simulink model "Clutchless_P2_Parallel_ETE"  (R2017b)
settings: Solver=FixedStepAuto  StartTime=0.0  StopTime=length(Speed)  FixedStep=0.01  MaxStep=0.01  RelTol=1e-3  EnableMultiTasking=on
PostLoadFcn:
  | , if any(exist('dsrtsu_mdlpostloadfcn', 'file') == [2, 3, 6]), try dsrtsu_mdlpostloadfcn('Execute', bdroot); catch fprintf('Error in PostLoadFcn (dsrtsu_mdlpostloadfcn) for model "%s":\n %s\n', bdroot, lasterr); end, end,
undefined symbols (not defined in the file): ABSEnable, Actuators, air, APP1_OOR, APP2_OOR, APP_Mismatch, Brk_Flt, cal, ClutchEngag, Clutchless_HSC_ETE, CS_On_Control, Driver, eng, Engine, EngOverTemp, ENGTRQ_MSMCH_Degraded_CP, ENGTRQ_MSMCH_ErrCritical_CP, ENGTRQ_MSMCH_LimpHome_CP, EngTrqMismatch, env, ess, ESSOverTemp, gb, KeyPos_Flt, KeyPosition, lib_Actuators, lib_Clutchless_HSC_ETE, lib_Driver, lib_EMachine_2017a, lib_Sensors_2017a, LossCAN, Machine, max_vehicle_rad_air_flow, MCUOverTemp, mot, MotDirMismatch, MotOverTemp, MotTrqMismatch, mph2ms, PRNDL_Flt, RegenBrkDisable, RegenFault, Sensors, ShiftLeverPosition, Speed, SW_CS_ON, SW_Engine_ON, t_amb, time, tloop
libraries: simulink x97, Pneumatic_lib x11, nesl_utility x9, EC2_libraries x7, powerlib_meascontrol x2, CalculationGallon x1, lib_Chassis x1, lib_DCDC x1, lib_Differential x1, lib_HVESS x1, fl_lib x1, lib_OBC x1
(part 1 of 9)
settings Model: DSRTSU_INTERNAL_RTI_VER=480  DSRTSU_INTERNAL_RTI_TYPE=rti1006  RTICANMMDATA=struct('GeneralSetupData',struct('modelroot','D:\EcoCAR3\Controls\HIL\Y3\P2_Parallel_MIL_Model','generalsettings',struct('filesettings',struct('destfolder',struct('Name','RTICANMM_FILES','Check',1),'buildfolder',struct('Name','.','Check',1),'AbsDestfolder',struct('Name','D:\EcoCAR3\Controls\HIL\Y3\P2_Parallel_MIL_Model\RTICANMM_FILES'),'AbsBuildfolder',struct('Name','D:\EcoCAR3\Controls\HIL\Y3\P2_Parallel_MIL_Model'))),'options',struct('addpaths',1,'rmpaths',1,'addtrcexclusion',logical(1),'cannavigator',struct('checkmonitoring',0),'show_usrtrc',0,'use_usrtrc',0),'advanced',struct('options',[1 1 1 1 1 1 1 1 1 1 1 1 1 1 1 1 1 1 1 1 1 1 1 1 1 1 1 1 1 1 1 1 1 1 1 1 1 1 1 1 1 1 1 1 1 1 1 1 1 1 1 1 1 1 1 1 1 1 1 1 1 1 1 1 1 1 1 1 1 1 1 1 1 1 1 1 1 1 1 1 1 1 1 1 1 1 1 1 1 1 1 1 1 1 1 1 1 1 1 1]),'MPSetup',{{}},'modelname','P2_Parallel_MIL_02_16_2017','block','P2_Parallel_MIL_02_16_2017'))  DSRTSU_INTERNAL_RTIFPGA=70  SimulationMode=accelerator  Creator=EcoCar  LastModifiedBy=Lyu19
settings SolverCC: ExtrapolationOrder=1  NumberNewtonIterations=4
settings OptimizationCC: BlockReduction=off  OptimizeBlockIOStorage=off  BufferReuse=off  GlobalBufferReuse=off  ExpressionFolding=off  LocalBlockOutputs=off  EfficientMapNaN2IntZero=off
settings DebuggingCC: AllowSymbolicDim=off  NonBusSignalsTreatedAsBus=warning  SFUnexpectedBacktrackingDiag=warning  SFNoUnconditionalDefaultTransitionDiag=warning  SFExecutionAtInitializationDiag=none
settings HardwareCC: ProdBitPerPointer=32  ProdBitPerSizeT=32  ProdBitPerPtrDiffT=32  ProdLargestAtomicInteger=Integer  ProdWordSize=32  ProdHWDeviceType=Custom Processor->Custom  TargetBitPerPointer=64  TargetBitPerSizeT=64  TargetBitPerPtrDiffT=64  TargetLongLongMode=on  TargetIntDivRoundTo=Zero  TargetEndianess=LittleEndian  TargetWordSize=64  TargetHWDeviceType=MATLAB Host  ProdEqTarget=off
settings ModelReferenceCC: PropagateSignalLabelsOutOfModel=off
settings CodeAppCC: MaxIdLength=128  StateflowObjectComments=on
settings GRTTargetCC: TargetLangStandard=C89/C90 (ANSI)  CombineOutputUpdateFcns=off  GRTInterface=on
settings ConfigComp: CovMetricSettings=dw  CovHtmlReporting=on  CovSaveCumulativeToWorkspaceVar=on  CovSaveSingleToWorkspaceVar=on  CovExternalEMLEnable=off
settings SimscapeCC: SimscapeNormalizeSystem=off

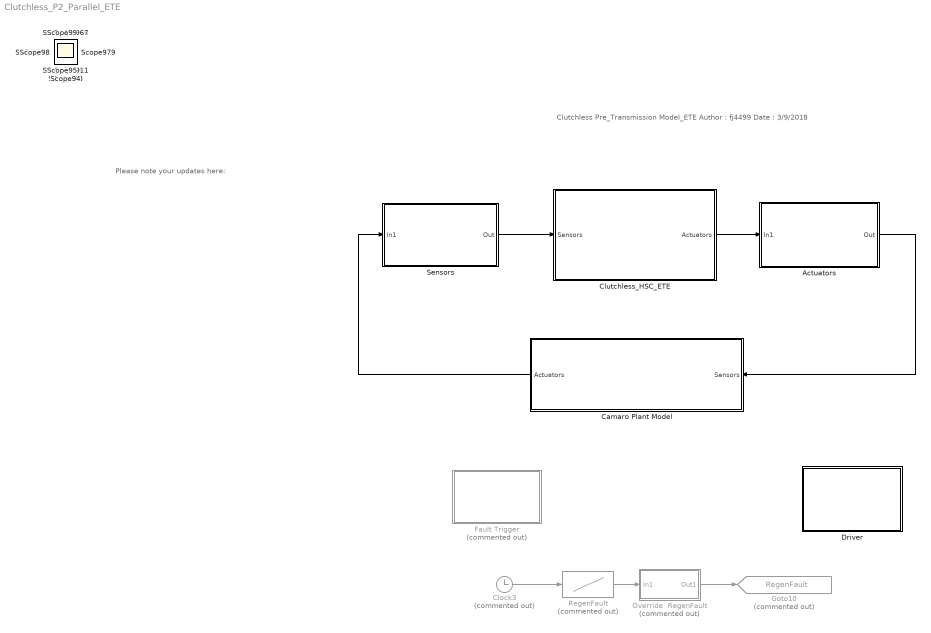
== system Clutchless_P2_Parallel_ETE ==
  note: Please note your updates here:
  note: Clutchless Pre_Transmission Model_ETE
      |
      | Author : fj4499
      | Date : 3/9/2018
  Actuators : Subsystem  AncestorBlock=lib_Actuators/Actuators
  Camaro Plant Model : Subsystem
      mask Display: image('Images/Vehicle.jpg')
  Clock3 : Clock  Commented=on
  Clutchless_HSC_ETE : Subsystem  AncestorBlock=lib_Clutchless_HSC_ETE/Clutchless_HSC_ETE
      mask Display: image('Images/HCU.jpg')
  Driver : Subsystem  AncestorBlock=lib_Driver/Driver
      mask Display: image('Images/Driver.jpg')
  "Fault Trigger " : Subsystem  Commented=on  mask(Fault Trigger){Mismatch_APP_ON=on, APP1_OOR_ON=on, APP2_OOR_ON=on, Brk_Flt_ON=on, KeyPos_Flt_ON=on, PRNDL_Flt_ON=on, LossCAN_ON=on, MotTrqMismatch_ON=on, MotDirMismatch_ON=on, EngTrqMismatch_ON=on, MotOverTemp_ON=on, MCUOverTemp_ON=on, EngOverTemp_ON=on, ESSOverTemp_ON=on, ClutchEngagFlt=on}
      mask help:
      | Check the box: override the fault (Control Port value=1;)
      | Uncheck the box: Implement the fault (Control Port value=0;)
      mask DialogControl DriverInterfaceFault Prompt: Driver Interface Fault
      mask DialogControl Container3 Prompt: Component Fault
      mask Display:
      | plot([1 2 2.01 3 4], [0 0 1 1 1]);
      | disp('           Fault Trigger')
  Goto10 : Goto  Commented=on  GotoTag=RegenFault  TagVisibility=global
  Override  RegenFault : Subsystem  Commented=on
  RegenFault : Lookup  Commented=on  InputValues=time  Table=RegenFault  LookUpMeth=Interpolation-Use End Values  OutDataTypeStr=int8
  Sensors : Subsystem  AncestorBlock=lib_Sensors_2017a/Sensors
  Scope{,1..141} (142 alike) : Scope
  wires:
  Clock3/1 -> RegenFault/1
  RegenFault/1 -> Override  RegenFault/1(In1)
  Override  RegenFault/1(Out1) -> Goto10/1
  Clutchless_HSC_ETE/1(Actuators) -> Actuators/1(In1)
  Actuators/1(Out) -> Camaro Plant Model/1(Sensors)
  Camaro Plant Model/1(Actuators) -> Sensors/1(In1)
  Sensors/1(Out) -> Clutchless_HSC_ETE/1(Sensors)

== system Clutchless_P2_Parallel_ETE/Actuators ==
  In1 : Inport
  Analog : Subsystem
  Bus Creator : BusCreator  Inputs=3
  CAN : Subsystem
  Digital : Subsystem
  Memory : Memory  InheritSampleTime=on
  Out : Outport
  wires:
  In1/1 -> CAN/1(In1), Analog/1(In1), Digital/1(In1)
  Bus Creator/1 -> Memory/1
  Digital/1(Out1) -> Bus Creator/3  "Digital"
  CAN/1(Out1) -> Bus Creator/1  "CAN"
  Analog/1(Out1) -> Bus Creator/2  "Analog"
  Memory/1 -> Out/1

== system Clutchless_P2_Parallel_ETE/Camaro Plant Model ==
  Sensors : Inport
  Add : Sum  Inputs=+++
      mask Display:
      | port_label('input',1,'+');
      | port_label('input',2,'+');
      | port_label('input',3,'+');
  Bus Creator : BusCreator  Inputs=3
  Bus Creator1 : BusCreator  Inputs=7
  Bus Creator2 : BusCreator  Inputs=1
  Bus Selector : BusSelector  OutputSignals=Analog,CAN.to VEH_CAN,CAN.to EBCAN,CAN.to HV_CAN,Digital
  Calculate MPGe : CalculationGallon/Calculate MPGe
  Chassis : lib_Chassis/Chassis  SystemSampleTime=-1
      link override Grade: InputValues=time
  DC-DC Converter : lib_DCDC/DC-DC Converter  SystemSampleTime=-1
  Differential : lib_Differential/Differential  SystemSampleTime=-1
      settings: SourceProductName=The database C:\Users\vrajm\AppData\Roaming\MathWorks\MATLAB\R2017b\slblocks_master.db is locked, or a table in the database is locked. (database is locked)
  E-Machine : Subsystem  AncestorBlock=lib_EMachine_2017a/E-Machine
      mask Display:
      | image('Images/motor.png')
      | color('red');
      | port_label('Input',1,'Volt');
      | port_label('Input',2,'ShaftIn');
      | port_label('Input',3,'SpdOut');
      | port_label('Output',1,'Crr');
      | port_label('Output',2,'ShaftOut');
      | port_label('Output',3,'SpdIn');
  ESS : lib_HVESS/ESS  SystemSampleTime=-1
  Ground : Ground
  ICE Simple1 : Subsystem  AncestorBlock=lib_Engine/ICE Simple1
      mask Display:
      | image(imread('EngineTopLevel.jpg'),'center')
      | color('red');
      | port_label('input',1,'SpdOut')
      | port_label('output',1,'ShaftOut')
  On-Board Charger : lib_OBC/On-Board Charger  SystemSampleTime=-1
      settings: SourceProductName=The database C:\Users\vrajm\AppData\Roaming\MathWorks\MATLAB\R2017b\slblocks_master.db is locked, or a table in the database is locked. (database is locked)
  Scopes : Subsystem  Commented=on
      mask Display: image('Images/Scope.jpg')
  Scopes1 : Scope_new/Scopes1  SystemSampleTime=-1
  Transmission : lib_Transmission/Transmission  SystemSampleTime=-1
  Transmission Validation Results : Transmission_Validation/Transmission Validation Results  Commented=on  SystemSampleTime=-1
  Wheels : lib_Wheels/Wheels  SystemSampleTime=-1
      link override Grade: InputValues=time
      settings: SourceProductName=The database C:\Users\vrajm\AppData\Roaming\MathWorks\MATLAB\R2017b\slblocks_master.db is locked, or a table in the database is locked. (database is locked)
  Actuators : Outport
  tag scope: Analog=global, Digital=global, HCU_to_EBCAN=global, HCU_to_HV_CAN=global, HCU_to_VEH_CAN=global
  wires:
  Differential/1 -> Wheels/1
  Wheels/1 -> Chassis/1
  Chassis/1 -> Wheels/2
  Differential/2 -> Transmission/2
  Transmission/1 -> Differential/1
  ESS/1 -> DC-DC Converter/1, E-Machine/1(voltage), On-Board Charger/1
  DC-DC Converter/1 -> Add/3
  On-Board Charger/1 -> Add/2
  Add/1 -> ESS/1
  Transmission/2 -> E-Machine/3(Mot_SpdOut)
  E-Machine/2(Motor_ShaftOut) -> Transmission/1
  E-Machine/1(current) -> Add/1
  Bus Creator/1 -> Actuators/1
  Sensors/1 -> Bus Selector/1
  Bus Selector/1 -> [Analog]  "<Analog>"
  Bus Selector/2 -> [HCU_to_VEH_CAN]  "<to VEH_CAN>"
  Bus Selector/3 -> [HCU_to_EBCAN]  "<to EBCAN>"
  Bus Selector/4 -> [HCU_to_HV_CAN]  "<to HV_CAN>"
  Bus Selector/5 -> [Digital]  "<Digital>"
  Wheels/2 -> Differential/2
  E-Machine/3(Motor_SpdIn) -> ICE Simple1/1(eng_spd_out)
  [ECM_to_HCU] -> Bus Creator1/1
  [TCM_to_HCU] -> Bus Creator1/2
  [BCM_to_HCU] -> Bus Creator1/3
  [BMS_to_HCU] -> Bus Creator1/4
  [MCU_to_HCU] -> Bus Creator1/5
  Bus Creator2/1 -> Bus Creator1/6  "APM_to_HCU"
  [OBC_to_HCU] -> Bus Creator1/7
  Bus Creator1/1 -> Bus Creator/1  "CAN"
  [Driver_Request] -> Bus Creator/2  "Driver_Signals"
  [DCDC_to_HCU] -> Bus Creator/3
  Ground/1 -> Bus Creator2/1  "APM_CAN"
  ICE Simple1/1(eng_shaft_out) -> E-Machine/2(Mot_ShaftIn)

== system Clutchless_P2_Parallel_ETE/Clutchless_HSC_ETE ==
  Sensors : Inport
  HSC : Subsystem
  Actuators : Outport
  wires:
  Sensors/1 -> HSC/1(Sensors)
  HSC/1(Actuators) -> Actuators/1

== system Clutchless_P2_Parallel_ETE/Driver ==
  Bus Creator : BusCreator  Inputs=12
  Bus Selector : BusSelector  OutputSignals=GFD_Light,HV_Chg_Light,Veh_Ready_Light
  Constant : Constant  Commented=on  Value=0
  Display : Display
  Display1 : Display
  Display2 : Display
  Driver Control : Subsystem
  Manual Control : Subsystem  Commented=on
  Multiport Switch1 : MultiPortSwitch  Commented=on  DataPortOrder=Zero-based contiguous  Inputs=2
  Subsystem : Subsystem
  tag scope: Driver_Request=global
  wires:
  Driver Control/11(Sport_Mode_SW) -> Bus Creator/12  "Sport_Mode_SW"
  Driver Control/10(ABS_Active) -> Bus Creator/11  "ABSAtv"
  Subsystem/2(APP2) -> Bus Creator/3
  Subsystem/1(APP1) -> Bus Creator/2
  Bus Selector/3 -> Display2/1  "<Veh_Ready_Light>"
  Bus Selector/2 -> Display1/1  "<HV_Chg_Light>"
  Bus Selector/1 -> Display/1  "<GFD_Light>"
  [Digital] -> Bus Selector/1
  Driver Control/9(CS_On) -> Bus Creator/10  "SW_CS_ON"
  Driver Control/8(Engine_On) -> Bus Creator/9  "SW_Engine_ON"
  Driver Control/7(Regen_Disable) -> Bus Creator/8  "SW_Regen_Disable"
  Driver Control/6(Veh_Spd) -> Bus Creator/7  "Veh_Spd"
  Bus Creator/1 -> [Driver_Request]
  Manual Control/1(Out1) -> Multiport Switch1/3
  Constant/1 -> Multiport Switch1/1
  Driver Control/5(EVSE_Pluggin) -> Bus Creator/6  "EVSE_Plugged"
  Driver Control/4(Shift Lever Position) -> Bus Creator/5  "ShiftLvrPos"
  Driver Control/3(BPP[%]) -> Bus Creator/4  "drv_BPP_req_[%]"
  Driver Control/2(APP[%]) -> Subsystem/1(In1)  "drv_APP_req_[%]"
  Driver Control/1(Key Position) -> Bus Creator/1  "KeyPos"

== system Clutchless_P2_Parallel_ETE/Fault Trigger  ==
  Clock3 : Clock
  Component Diagnostics setting : Subsystem
  Driver Interface Diagnostics setting : Subsystem
  wires:
  Clock3/1 -> Component Diagnostics setting/1(time), Driver Interface Diagnostics setting/1(time)

== system Clutchless_P2_Parallel_ETE/Override  RegenFault ==
  note: This subsystem is used to override the model value of a signal to a constant value
  note: Override Switch Subsystem
  In1 : Inport
  Constant : Constant  Value=0
  Multiport Switch : MultiPortSwitch  DataPortOrder=Zero-based contiguous  Inputs=2
  Signal Override Switch 0 = Use Model 1 = Use Constant : Constant  Value=0
  Out1 : Outport
  wires:
  Signal Override Switch 0 = Use Model 1 = Use Constant/1 -> Multiport Switch/1
  In1/1 -> Multiport Switch/2
  Multiport Switch/1 -> Out1/1
  Constant/1 -> Multiport Switch/3

== system Clutchless_P2_Parallel_ETE/Sensors ==
  In1 : Inport
  Analog : Subsystem
  Bus Creator : BusCreator  Inputs=3
  Bus Selector : BusSelector  OutputSignals=CAN
  CAN : Subsystem
  Digital : Subsystem
  Out : Outport
  wires:
  Bus Creator/1 -> Out/1
  In1/1 -> Digital/1(In1), Analog/1(In1), Bus Selector/1
  Bus Selector/1 -> CAN/1(In1)  "<CAN>"
  CAN/1(Out1) -> Bus Creator/1  "from_CAN"
  Analog/1(Out1) -> Bus Creator/2  "from_Analog"
  Digital/1(Out1) -> Bus Creator/3  "from_Digital"

== system Clutchless_P2_Parallel_ETE/Actuators/Analog ==
  In1 : Inport
  Bus Creator : BusCreator  Inputs=1
  Bus Selector : BusSelector  OutputSignals=Controls.EngAppReq
  Data Type Conversion : DataTypeConversion
  Out1 : Outport
  wires:
  In1/1 -> Bus Selector/1
  Bus Creator/1 -> Out1/1
  Bus Selector/1 -> Data Type Conversion/1  "<EngAppReq>"
  Data Type Conversion/1 -> Bus Creator/1  "EngAppReq"

== system Clutchless_P2_Parallel_ETE/Actuators/CAN ==
  In1 : Inport
  Bus Creator : BusCreator  Inputs=3
  EBCAN : Subsystem
  HV_CAN : Subsystem
  VEH_CAN : Subsystem
  Out1 : Outport
  wires:
  VEH_CAN/1(Out1) -> Bus Creator/1  "to VEH_CAN"
  EBCAN/1(Out1) -> Bus Creator/2  "to EBCAN"
  HV_CAN/1(Out1) -> Bus Creator/3  "to HV_CAN"
  Bus Creator/1 -> Out1/1
  In1/1 -> HV_CAN/1(In1), EBCAN/1(In1), VEH_CAN/1(In1)

== system Clutchless_P2_Parallel_ETE/Actuators/Digital ==
  In1 : Inport
  Bus Creator : BusCreator  Inputs=8
  Bus Selector : BusSelector  OutputSignals=BMS_Digital.T_15,BMS_Digital.T_30,BMS_Digital.T_30C,Fuel_Pump_Control.Pump_Commands.FuelPump_Disable,OBC_Digital.Brusa_Enable,Axiomatic_CAN.GFD_Light,Axiomatic_CAN.HV_Chg_Light,Axiomatic_CAN.Veh_Ready_Light
  Data Type Conversion : DataTypeConversion
  Data Type Conversion1 : DataTypeConversion
  Out1 : Outport
  wires:
  In1/1 -> Bus Selector/1
  Bus Creator/1 -> Out1/1  "Digital"
  Bus Selector/4 -> Bus Creator/4  "<FuelPump_Disable>"
  Bus Selector/3 -> Bus Creator/3  "<T_30C>"
  Bus Selector/2 -> Data Type Conversion1/1  "<T_30>"
  Bus Selector/1 -> Data Type Conversion/1  "<T_15>"
  Bus Selector/5 -> Bus Creator/5  "<Brusa_Enable>"
  Bus Selector/6 -> Bus Creator/6  "<GFD_Light>"
  Bus Selector/7 -> Bus Creator/7  "<HV_Chg_Light>"
  Bus Selector/8 -> Bus Creator/8  "<Veh_Ready_Light>"
  Data Type Conversion/1 -> Bus Creator/1  "T_15"
  Data Type Conversion1/1 -> Bus Creator/2  "T_30"

== system Clutchless_P2_Parallel_ETE/Camaro Plant Model/E-Machine ==
  voltage : Inport
  Mot_ShaftIn : Inport  Port=2
  Mot_SpdOut : Inport  Port=3
  Clutch Temporary 1 : Subsystem  Commented=on
  IMG Plant : Subsystem
      mask Display:
      | image('Images\Motor.png')
      | color('red');
      | port_label('Input',2,'Volt');
      | port_label('Input',3,'ShaftIn');
      | port_label('Input',4,'SpdOut');
      | port_label('Output',2,'Crr');
      | port_label('Output',3,'ShaftOut');
      | port_label('Output',4,'SpdIn');
  IMG Plant2 : Subsystem  Commented=on
      mask Display:
      | image('Images/motor.png')
      | color('red');
      | port_label('Input',2,'Volt');
      | port_label('Input',3,'SpdOut');
      | port_label('Input',1,'MCU_cmd');
      | port_label('Input',4,'ShaftIn');
      | port_label('Output',1,'Sensor_Out');
      | port_label('Output',2,'Crr');
      | port_label('Output',3,'MotTrqOut');
      | port_label('Output',4,'MotSpdIn');
  Soft MCU : Subsystem
      mask Display: image('SoftECU.jpg')
  current : Outport
  Motor_ShaftOut : Outport  Port=2
  Motor_SpdIn : Outport  Port=3
  tag scope: MCU_to_HCU=global
  wires:
  IMG Plant/2(current) -> current/1
  voltage/1 -> IMG Plant/2(voltage)
  IMG Plant/3(MotShaftOut) -> Motor_ShaftOut/1
  Mot_ShaftIn/1 -> IMG Plant/3(MotShaftIn)
  IMG Plant/1(Out1) -> Soft MCU/2(In1)  "Sensors_to_MCU"
  [HCU_to_HV_CAN] -> Soft MCU/1(In)
  Soft MCU/2(Out1) -> IMG Plant/1("In1 ")  "MCU_to_Actuators"
  Soft MCU/1(Out) -> [MCU_to_HCU]
  Mot_SpdOut/1 -> IMG Plant/4(SpdOut)
  IMG Plant/4(SpdIn) -> Motor_SpdIn/1

== system Clutchless_P2_Parallel_ETE/Camaro Plant Model/ICE Simple1 ==
  eng_spd_out : Inport
  Engine Plant Modified : Subsystem
      mask Display:
      | image(imread('EngineTopLevel.jpg'),'center')
      | color('red');
      | port_label('input',2,'SpdOut')
      | port_label('output',2,'ShaftOut')
  Inputs : Subsystem
  Soft ECM : Subsystem
      mask Display: image('SoftECU.jpg')
  eng_shaft_out : Outport
  tag scope: ECM_to_HCU=global
  wires:
  Engine Plant Modified/2(Out) -> Soft ECM/2(In1)
  eng_spd_out/1 -> Engine Plant Modified/2(eng_spd_out)
  Soft ECM/2(Out1) -> Engine Plant Modified/1("In ")  "ECM_to_Actuators"
  Inputs/1(Inputs) -> Soft ECM/1(In)
  Soft ECM/1(Out) -> [ECM_to_HCU]
  Engine Plant Modified/1(eng_shaft_out) -> eng_shaft_out/1

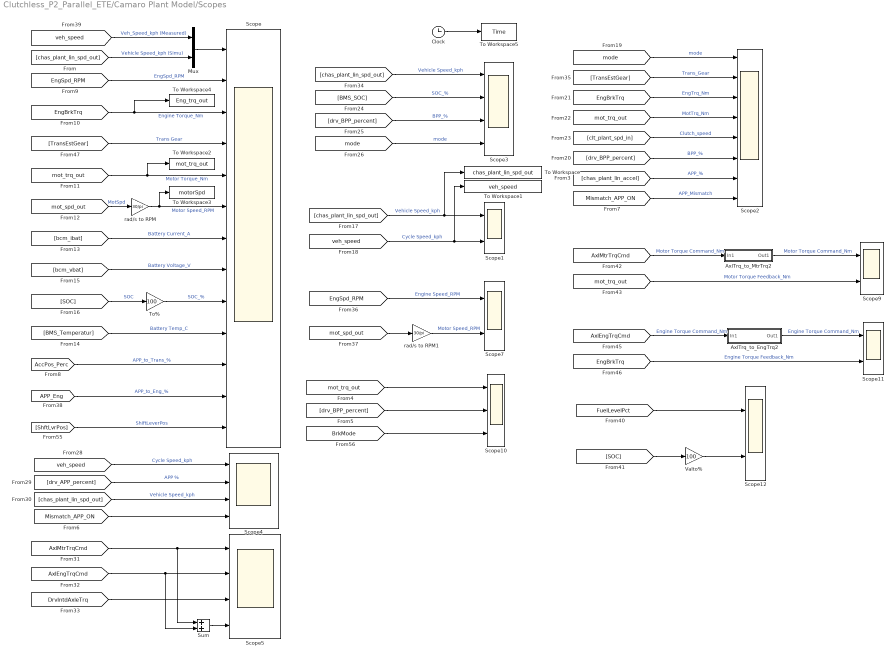
== system Clutchless_P2_Parallel_ETE/Camaro Plant Model/Scopes ==
  AxlTrq_to_EngTrq2 : Subsystem
  AxlTrq_to_MtrTrq2 : Subsystem
  Clock : Clock
      settings: Decimation=WORKSPACE_DECIMATION
  Mux : Mux  Inputs=2
  Scope : Scope  NumInputPorts=13
  Scope{1,7,9,11..12} (5 alike) : Scope  NumInputPorts=2
  Scope10 : Scope  NumInputPorts=3
  Scope2 : Scope  NumInputPorts=8
  Scope3 : Scope  NumInputPorts=4
  Scope4 : Scope  NumInputPorts=4
  Scope5 : Scope  NumInputPorts=4
  Sum : Sum
  To Workspace : ToWorkspace  VariableName=chas_plant_lin_spd_out  SampleTime=-1
  To Workspace1 : ToWorkspace  VariableName=veh_speed  SampleTime=-1
  To Workspace2 : ToWorkspace  VariableName=mot_trq_out  SampleTime=-1
  To Workspace3 : ToWorkspace  VariableName=motorSpd  SampleTime=-1
  To Workspace4 : ToWorkspace  VariableName=Eng_trq_out  SampleTime=-1
  To Workspace5 : ToWorkspace  VariableName=Time  SampleTime=-1
      settings: Decimation=WORKSPACE_DECIMATION
  To% : Gain  Gain=100
  Valto% : Gain  Gain=100
  rad/s to RPM : Gain  Gain=30/pi
  rad/s to RPM1 : Gain  Gain=30/pi
  wires:
  [chas_plant_lin_spd_out] -> Mux/2  "Vehicle Speed_kph (Simu)"
  [EngSpd_RPM] -> Scope/2  "EngSpd_RPM"
  [EngBrkTrq] -> To Workspace4/1, Scope/3  "Engine Torque_Nm"
  [mot_spd_out] -> rad/s to RPM/1  "MotSpd"
  [BMS_Temperatur] -> Scope/10  "Battery Temp_C"
  rad/s to RPM/1 -> To Workspace3/1, Scope/6  "Motor Speed_RPM"
  [mot_trq_out] -> To Workspace2/1, Scope/5  "Motor Torque_Nm"
  To%/1 -> Scope/9  "SOC_%"
  [TransEstGear] -> Scope/4  "Trans Gear"
  [bcm_ibat] -> Scope/7  "Battery Current_A"
  [chas_plant_lin_spd_out] -> Scope3/1  "Vehicle Speed_kph"
  [BMS_SOC] -> Scope3/2  "SOC_%"
  [drv_BPP_percent] -> Scope3/3  "BPP_%"
  [mode] -> Scope3/4  "mode"
  [chas_plant_lin_spd_out] -> To Workspace/1, Scope1/1  "Vehicle Speed_kph"
  [veh_speed] -> To Workspace1/1, Scope1/2  "Cycle Speed_kph"
  [mode] -> Scope2/1  "mode"
  [EngBrkTrq] -> Scope2/3  "EngTrq_Nm"
  [mot_trq_out] -> Scope2/4  "MotTrq_Nm"
  [clt_plant_spd_in] -> Scope2/5  "Clutch_speed"
  [EngSpd_RPM] -> Scope7/1  "Engine Speed_RPM"
  [mot_spd_out] -> rad/s to RPM1/1
  rad/s to RPM1/1 -> Scope7/2  "Motor Speed_RPM"
  [veh_speed] -> Scope4/1  "Cycle Speed_kph"
  [drv_APP_percent] -> Scope4/2  "APP %"
  [chas_plant_lin_spd_out] -> Scope4/3  "Vehicle Speed_kph"
  [AxlMtrTrqCmd] -> Sum/1, Scope5/1
  [AxlEngTrqCmd] -> Sum/2, Scope5/2
  [DrvIntdAxleTrq] -> Scope5/3
  Sum/1 -> Scope5/4
  [AxlMtrTrqCmd] -> AxlTrq_to_MtrTrq2/1(In1)  "Motor Torque Command_Nm"
  [mot_trq_out] -> Scope9/2  "Motor Torque Feedback_Nm"
  [AxlEngTrqCmd] -> AxlTrq_to_EngTrq2/1(In1)  "Engine Torque Command_Nm"
  [EngBrkTrq] -> Scope11/2  "Engine Torque Feedback_Nm"
  [TransEstGear] -> Scope2/2  "Trans_Gear"
  [drv_BPP_percent] -> Scope2/6  "BPP_%"
  [chas_plant_lin_accel] -> Scope2/7  "APP_%"
  AxlTrq_to_MtrTrq2/1(Out1) -> Scope9/1  "Motor Torque Command_Nm"
  AxlTrq_to_EngTrq2/1(Out1) -> Scope11/1  "Engine Torque Command_Nm"
  [bcm_vbat] -> Scope/8  "Battery Voltage_V"
  [Mismatch_APP_ON] -> Scope4/4
  [Mismatch_APP_ON] -> Scope2/8  "APP_Mismatch"
  [SOC] -> To%/1  "SOC"
  [AccPos_Perc] -> Scope/11  "APP_to_Trans_%"
  [APP_Eng] -> Scope/12  "APP_to_Eng_%"
  Mux/1 -> Scope/1
  [veh_speed] -> Mux/1  "Veh_Speed_kph (Measured)"
  Clock/1 -> To Workspace5/1
  [FuelLevelPct] -> Scope12/1
  [SOC] -> Valto%/1
  Valto%/1 -> Scope12/2
  [ShftLvrPos] -> Scope/13  "ShiftLeverPos"
  [mot_trq_out] -> Scope10/1
  [drv_BPP_percent] -> Scope10/2
  [BrkMode] -> Scope10/3

== system Clutchless_P2_Parallel_ETE/Clutchless_HSC_ETE/HSC ==
  Sensors : Inport
  Camaro Fault Detection : Subsystem
  Driver_Requests : Subsystem  RequirementInfo={} %GIDa_ee5d0f02_0a71_4952_8ea3_2a40744828e3
  Powertrain Manager : Subsystem
  Actuators : Outport
  wires:
  Powertrain Manager/2(Controls) -> Driver_Requests/3("Controls ")
  Sensors/1 -> Camaro Fault Detection/1(Sensors), Powertrain Manager/1(Sensors), Driver_Requests/1(Sensors)
  Powertrain Manager/1(Out1) -> Actuators/1
  Camaro Fault Detection/1(Diagnostic) -> Powertrain Manager/3(Fault Detection), Driver_Requests/2("Diagnostic ")
  Driver_Requests/1(DriverRequests) -> Powertrain Manager/2(Driver Request)

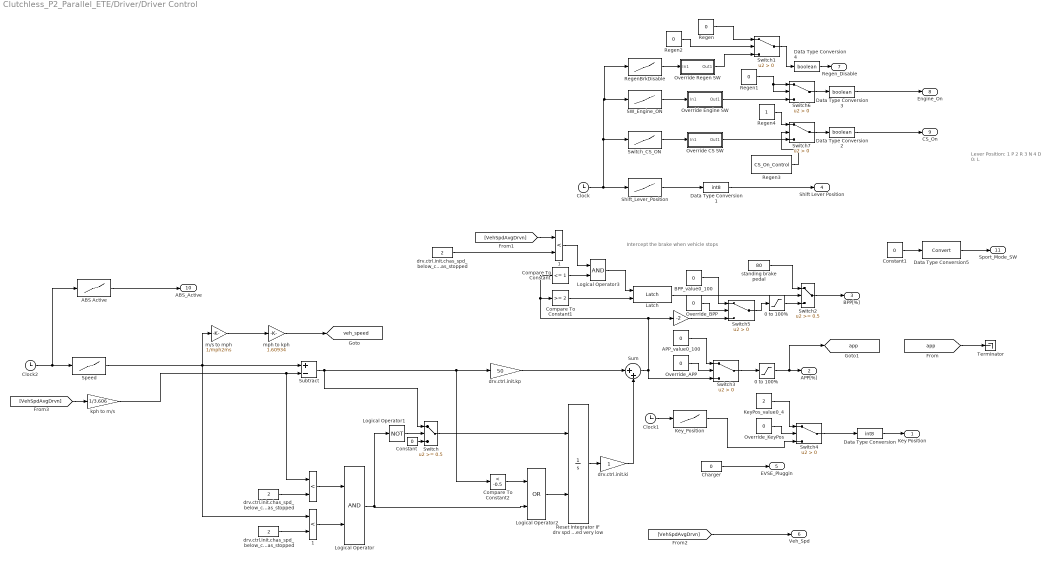
== system Clutchless_P2_Parallel_ETE/Driver/Driver Control ==
  note: Intercept the brake when vehicle stops
  note: Lever Position:
      | 1 P
      | 2 R
      | 3 N
      | 4 D
      | 0: L
  " " : Gain  Gain=-2
  "    " : RelationalOperator  Operator=<  RndMeth=Nearest  InputSameDT=on
  "    1" : RelationalOperator  Operator=<  RndMeth=Nearest  InputSameDT=on
  "  1" : RelationalOperator  Operator=<  RndMeth=Nearest  InputSameDT=on
  0 to 100% : Saturate  UpperLimit=100  LowerLimit=0
  "0 to 100% " : Saturate  UpperLimit=100  LowerLimit=0
  ABS Active : Lookup  InputValues=time  Table=ABSEnable
  APP_value0_100 : Constant  Value=0
  BPP_value0_100 : Constant  Value=0
  Charger : Constant  Value=0
  Clock : Clock
  Clock1 : Clock
  Clock2 : Clock
  Compare To Constant : simulink/Logic and Bit Operations/Compare To Constant  relop=<=  const=1  OutDataTypeStr=boolean
  Compare To Constant1 : simulink/Logic and Bit Operations/Compare To Constant  relop=>=  const=2  OutDataTypeStr=boolean
  Compare To Constant2 : simulink/Logic and Bit Operations/Compare To Constant  relop=<  const=-0.5  OutDataTypeStr=boolean
  Constant : Constant  Value=0
  Constant1 : Constant  Value=0
  Data Type Conversion : DataTypeConversion  OutDataTypeStr=int8
  Data Type Conversion1 : DataTypeConversion  OutDataTypeStr=int8
  Data Type Conversion2 : DataTypeConversion  OutDataTypeStr=boolean
  Data Type Conversion3 : DataTypeConversion  OutDataTypeStr=boolean
  Data Type Conversion4 : DataTypeConversion  OutDataTypeStr=boolean
  Data Type Conversion5 : DataTypeConversion
  KeyPos_value0_4 : Constant  Value=2
  Key_Position : Lookup  InputValues=time  Table=KeyPosition
  Latch : Utility/Latch
  Logical Operator : Logic  AllPortsSameDT=off  OutDataTypeStr=boolean
  Logical Operator1 : Logic  Operator=NOT  AllPortsSameDT=off  OutDataTypeStr=boolean
  Logical Operator2 : Logic  Operator=OR  AllPortsSameDT=off  OutDataTypeStr=boolean
  Logical Operator3 : Logic  AllPortsSameDT=off  OutDataTypeStr=boolean
  Override CS SW : Subsystem
  Override Engine SW : Subsystem
  Override Regen SW : Subsystem
  Override_APP : Constant  Value=0
  Override_BPP : Constant  Value=0
  Override_KeyPos : Constant  Value=0
  Regen : Constant  Value=0
  Regen1 : Constant  Value=0
  Regen2 : Constant  Value=0
  Regen3 : Constant  Value=CS_On_Control
  Regen4 : Constant
  RegenBrkDisable : Lookup  InputValues=time  Table=RegenBrkDisable
  Reset Integrator IF drv spd dmd very low AND AND current vehicle speed very low : Integrator  ExternalReset=either
  SW_Engine_ON : Lookup  InputValues=time  Table=SW_Engine_ON
  Shift_Lever_Position : Lookup  InputValues=time  Table=ShiftLeverPosition
  Speed : Lookup  InputValues=time  Table=Speed
  Subtract : Sum  Inputs=+-
  Sum : Sum  Inputs=|++  SaturateOnIntegerOverflow=on  InputSameDT=on  OutDataTypeStr=Inherit: Same as first input
  Switch : Switch  Threshold=0.5
  Switch{1,3..7} (6 alike) : Switch  Criteria=u2 > Threshold
  Switch2 : Switch  Threshold=0.5
  Switch_CS_ON : Lookup  InputValues=time  Table=SW_CS_ON
  Terminator : Terminator
  "drv.ctrl.init.chas_spd_below_chas_stopped " : Constant  Value=2
  "drv.ctrl.init.chas_spd_below_chas_stopped " : Constant  Value=2
  "drv.ctrl.init.chas_spd_below_chas_stopped " : Constant  Value=2
  drv.ctrl.init.ki : Gain  SaturateOnIntegerOverflow=on  OutDataTypeStr=Inherit: Same as input  ParamDataTypeStr=Inherit: Same as input
  drv.ctrl.init.kp : Gain  Gain=50  SaturateOnIntegerOverflow=on  OutDataTypeStr=Inherit: Same as input  ParamDataTypeStr=Inherit: Same as input
  kph to m/s : Gain  Gain=1/3.606  SaturateOnIntegerOverflow=on  OutDataTypeStr=Inherit: Same as input  ParamDataTypeStr=Inherit: Same as input
  m/s to mph : Gain  Gain=1/mph2ms
  mph to kph : Gain  Gain=1.60934
  standing brake pedal : Constant  Value=80
  Key Position : Outport
  APP[%] : Outport  Port=2
  BPP[%] : Outport  Port=3
  Shift Lever Position : Outport  Port=4
  EVSE_Pluggin : Outport  Port=5
  Veh_Spd : Outport  Port=6
  Regen_Disable : Outport  Port=7
  Engine_On : Outport  Port=8
  CS_On : Outport  Port=9
  ABS_Active : Outport  Port=10
  Sport_Mode_SW : Outport  Port=11
  tag scope: app=global, veh_speed=global
  wires:
  Speed/1 -> "  1"/1, m/s to mph/1, Subtract/1
  [app] -> Terminator/1
  Regen4/1 -> Switch7/1
  Regen3/1 -> Switch7/2
  Override CS SW/1(Out1) -> Switch7/3
  Switch7/1 -> Data Type Conversion2/1
  Regen2/1 -> Switch1/2
  Constant1/1 -> Data Type Conversion5/1
  Data Type Conversion5/1 -> Sport_Mode_SW/1
  ABS Active/1 -> ABS_Active/1
  kph to m/s/1 -> "    "/1, Subtract/2
  Switch6/1 -> Data Type Conversion3/1
  Override Engine SW/1(Out1) -> Switch6/3
  Data Type Conversion3/1 -> Engine_On/1
  Regen1/1 -> Switch6/1, Switch6/2
  Switch1/1 -> Data Type Conversion4/1
  Regen/1 -> Switch1/1
  Shift_Lever_Position/1 -> Data Type Conversion1/1
  Switch5/1 -> "0 to 100% "/1
  BPP_value0_100/1 -> Switch5/1
  Override_BPP/1 -> Switch5/2
  Latch/1 -> Switch2/2
  Switch4/1 -> Data Type Conversion/1
  KeyPos_value0_4/1 -> Switch4/1
  Override_KeyPos/1 -> Switch4/2
  Key_Position/1 -> Switch4/3
  APP_value0_100/1 -> Switch3/1
  Override_APP/1 -> Switch3/2
  Switch3/1 -> 0 to 100%/1
  [VehSpdAvgDrvn] -> Veh_Spd/1
  Data Type Conversion4/1 -> Regen_Disable/1
  Data Type Conversion2/1 -> CS_On/1
  Override Regen SW/1(Out1) -> Switch1/3
  RegenBrkDisable/1 -> Override Regen SW/1(In1)
  SW_Engine_ON/1 -> Override Engine SW/1(In1)
  Switch_CS_ON/1 -> Override CS SW/1(In1)
  0 to 100%/1 -> APP[%]/1, [app]
  mph to kph/1 -> [veh_speed]
  m/s to mph/1 -> mph to kph/1
  Clock2/1 -> Speed/1, ABS Active/1
  Clock1/1 -> Key_Position/1
  Clock/1 -> Shift_Lever_Position/1, Switch_CS_ON/1, SW_Engine_ON/1, RegenBrkDisable/1
  Compare To Constant2/1 -> Logical Operator2/1
  Subtract/1 -> Switch/1, drv.ctrl.init.kp/1, Compare To Constant2/1
  Charger/1 -> EVSE_Pluggin/1
  Data Type Conversion1/1 -> Shift Lever Position/1
  Data Type Conversion/1 -> Key Position/1
  Compare To Constant1/1 -> Latch/2
  Compare To Constant/1 -> Logical Operator3/2
  Logical Operator3/1 -> Latch/1
  Sum/1 -> Switch3/3, " "/1, Compare To Constant/1, Compare To Constant1/1
  "    1"/1 -> Logical Operator3/1
  "drv.ctrl.init.chas_spd_below_chas_stopped "/1 -> "    1"/2
  [VehSpdAvgDrvn] -> "    1"/1
  Switch2/1 -> BPP[%]/1
  standing brake pedal/1 -> Switch2/1
  [VehSpdAvgDrvn] -> kph to m/s/1
  " "/1 -> Switch5/3
  "0 to 100% "/1 -> Switch2/3
  Logical Operator/1 -> Logical Operator1/1, Logical Operator2/2
  "  1"/1 -> Logical Operator/2
  drv.ctrl.init.ki/1 -> Sum/2
  "drv.ctrl.init.chas_spd_below_chas_stopped "/1 -> "  1"/2
  Logical Operator2/1 -> Reset Integrator IF drv spd dmd very low AND AND current vehicle speed very low/2
  Switch/1 -> Reset Integrator IF drv spd dmd very low AND AND current vehicle speed very low/1
  "drv.ctrl.init.chas_spd_below_chas_stopped "/1 -> "    "/2
  Logical Operator1/1 -> Switch/2
  Reset Integrator IF drv spd dmd very low AND AND current vehicle speed very low/1 -> drv.ctrl.init.ki/1
  Constant/1 -> Switch/3
  "    "/1 -> Logical Operator/1
  drv.ctrl.init.kp/1 -> Sum/1

== system Clutchless_P2_Parallel_ETE/Driver/Manual Control ==
  note: Manipulate these values
      | to drive vehicle
  APP[%] : Constant
  BPP[%] : Constant  Value=-1
  Bus Creator1 : BusCreator  Inputs=5
  KeyPosition : Constant  Value=3
  PRNDL : Constant  Value=4
  ReferenceVel1 : Constant  Value=0
  Saturation : Saturate  UpperLimit=100  LowerLimit=0
  Saturation1 : Saturate  UpperLimit=0  LowerLimit=-100
  Saturation2 : Saturate  UpperLimit=3  LowerLimit=0
  Saturation3 : Saturate  UpperLimit=4  LowerLimit=0
  Slider Gain : simulink/Math Operations/Slider Gain  gain=0  low=0  high=100
  Slider Gain1 : simulink/Math Operations/Slider Gain  gain=0  low=0  high=100
  Out1 : Outport
  wires:
  Slider Gain1/1 -> Saturation1/1
  Slider Gain/1 -> Saturation/1
  Saturation3/1 -> Bus Creator1/4  "PRNDL"
  PRNDL/1 -> Saturation3/1
  ReferenceVel1/1 -> Bus Creator1/5  "refVel [m/s]"
  APP[%]/1 -> Slider Gain/1
  BPP[%]/1 -> Slider Gain1/1
  Bus Creator1/1 -> Out1/1  "DriverOut"
  KeyPosition/1 -> Saturation2/1
  Saturation/1 -> Bus Creator1/1  "APP (%)"
  Saturation1/1 -> Bus Creator1/2  "BPP(%)"
  Saturation2/1 -> Bus Creator1/3  "Key_Pos_[0_3]"

== system Clutchless_P2_Parallel_ETE/Driver/Subsystem ==
  In1 : Inport
  Add1 : Sum  Inputs=+++
  Add2 : Sum
  Constant1 : Constant  Value=0
  Constant2 : Constant  Value=cal.APP.Mismatch_Value+0.1
  Constant3 : Constant  Value=0
  Constant4 : Constant  Value=cal.APP2.IN_Max_SC_Prcnt+1
  Constant5 : Constant  Value=0
  Constant6 : Constant  Value=cal.APP2.IN_Max_SC_Prcnt+1
  Switch : Switch  Threshold=1
  Switch1 : Switch  Threshold=1
  Switch2 : Switch  Threshold=1
  APP1 : Outport
  APP2 : Outport  Port=2
  wires:
  Switch2/1 -> Add2/2
  Add2/1 -> APP1/1  "drv_APP1"
  [APP2_OOR_ON] -> Switch2/2
  Constant6/1 -> Switch2/1
  Constant5/1 -> Switch2/3
  In1/1 -> Add1/1, Add2/1
  Add1/1 -> APP2/1  "drv_APP2"
  Switch1/1 -> Add1/3
  [APP2_OOR_ON] -> Switch1/2
  Constant4/1 -> Switch1/1
  Constant3/1 -> Switch1/3
  Constant2/1 -> Switch/1
  Constant1/1 -> Switch/3
  Switch/1 -> Add1/2
  [Mismatch_APP_ON] -> Switch/2

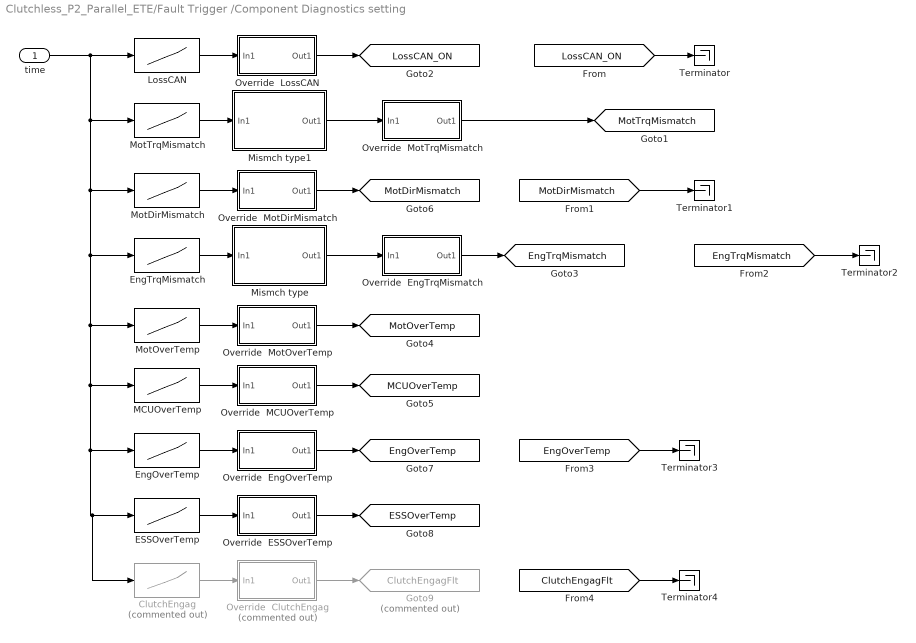
== system Clutchless_P2_Parallel_ETE/Fault Trigger /Component Diagnostics setting ==
  time : Inport
  ClutchEngag : Lookup  Commented=on  InputValues=time  Table=ClutchEngag  LookUpMeth=Interpolation-Use End Values  OutDataTypeStr=int8
  ESSOverTemp : Lookup  InputValues=time  Table=ESSOverTemp  LookUpMeth=Interpolation-Use End Values  OutDataTypeStr=int8
  EngOverTemp : Lookup  InputValues=time  Table=EngOverTemp  LookUpMeth=Interpolation-Use End Values  OutDataTypeStr=int8
  EngTrqMismatch : Lookup  InputValues=time  Table=EngTrqMismatch  LookUpMeth=Interpolation-Use End Values  OutDataTypeStr=int8
  Goto9 : Goto  Commented=on  GotoTag=ClutchEngagFlt  TagVisibility=global
  LossCAN : Lookup  InputValues=time  Table=LossCAN  LookUpMeth=Interpolation-Use End Values  OutDataTypeStr=int8
  MCUOverTemp : Lookup  InputValues=time  Table=MCUOverTemp  LookUpMeth=Interpolation-Use End Values  OutDataTypeStr=int8
  Mismch type : Subsystem
  Mismch type1 : Subsystem
  MotDirMismatch : Lookup  InputValues=time  Table=MotDirMismatch  LookUpMeth=Interpolation-Use End Values  OutDataTypeStr=int8
  MotOverTemp : Lookup  InputValues=time  Table=MotOverTemp  LookUpMeth=Interpolation-Use End Values  OutDataTypeStr=int8
  MotTrqMismatch : Lookup  InputValues=time  Table=MotTrqMismatch  LookUpMeth=Interpolation-Use End Values  OutDataTypeStr=int8
  Override  ClutchEngag : Subsystem  Commented=on
  Override  ESSOverTemp : Subsystem
  Override  EngOverTemp : Subsystem
  Override  EngTrqMismatch : Subsystem
  Override  LossCAN : Subsystem
  Override  MCUOverTemp : Subsystem
  Override  MotDirMismatch : Subsystem
  Override  MotOverTemp : Subsystem
  Override  MotTrqMismatch : Subsystem
  Terminator{,1..4} (5 alike) : Terminator
  tag scope: ESSOverTemp=global, EngOverTemp=global, EngTrqMismatch=global, LossCAN_ON=global, MCUOverTemp=global, MotDirMismatch=global, MotOverTemp=global, MotTrqMismatch=global
  wires:
  MotOverTemp/1 -> Override  MotOverTemp/1(In1)
  LossCAN/1 -> Override  LossCAN/1(In1)
  time/1 -> LossCAN/1, MotTrqMismatch/1, EngTrqMismatch/1, MotOverTemp/1, MCUOverTemp/1, EngOverTemp/1, ClutchEngag/1, ESSOverTemp/1, MotDirMismatch/1
  Override  LossCAN/1(Out1) -> [LossCAN_ON]
  Override  MCUOverTemp/1(Out1) -> [MCUOverTemp]
  Override  EngTrqMismatch/1(Out1) -> [EngTrqMismatch]
  Override  MotDirMismatch/1(Out1) -> [MotDirMismatch]
  MotDirMismatch/1 -> Override  MotDirMismatch/1(In1)
  Override  MotTrqMismatch/1(Out1) -> [MotTrqMismatch]
  MotTrqMismatch/1 -> Mismch type1/1(In1)
  EngTrqMismatch/1 -> Mismch type/1(In1)
  Override  MotOverTemp/1(Out1) -> [MotOverTemp]
  MCUOverTemp/1 -> Override  MCUOverTemp/1(In1)
  Override  EngOverTemp/1(Out1) -> [EngOverTemp]
  EngOverTemp/1 -> Override  EngOverTemp/1(In1)
  Override  ESSOverTemp/1(Out1) -> [ESSOverTemp]
  ESSOverTemp/1 -> Override  ESSOverTemp/1(In1)
  Override  ClutchEngag/1(Out1) -> Goto9/1
  ClutchEngag/1 -> Override  ClutchEngag/1(In1)
  Mismch type/1(Out1) -> Override  EngTrqMismatch/1(In1)
  Mismch type1/1(Out1) -> Override  MotTrqMismatch/1(In1)
  [LossCAN_ON] -> Terminator/1
  [MotDirMismatch] -> Terminator1/1
  [EngTrqMismatch] -> Terminator2/1
  [EngOverTemp] -> Terminator3/1
  [ClutchEngagFlt] -> Terminator4/1

== system Clutchless_P2_Parallel_ETE/Fault Trigger /Driver Interface Diagnostics setting ==
  time : Inport
  APP1_OOR : Lookup  InputValues=time  Table=APP1_OOR  LookUpMeth=Interpolation-Use End Values  OutDataTypeStr=int8
  APP2_OOR : Lookup  InputValues=time  Table=APP2_OOR  LookUpMeth=Interpolation-Use End Values  OutDataTypeStr=int8
  APP_Mismatch : Lookup  InputValues=time  Table=APP_Mismatch  LookUpMeth=Interpolation-Use End Values  OutDataTypeStr=int8
  BPP_Flt : Lookup  InputValues=time  Table=Brk_Flt  LookUpMeth=Interpolation-Use End Values  OutDataTypeStr=int8
  KeyPos_Flt : Lookup  InputValues=time  Table=KeyPos_Flt  LookUpMeth=Interpolation-Use End Values  OutDataTypeStr=int8
  Override  APP1_OOR : Subsystem
  Override  APP2_OOR : Subsystem
  Override  APP_Mismatch : Subsystem
  Override  BPP_Flt : Subsystem
  Override  KeyPos_Flt : Subsystem
  Override  PRNDL_Flt : Subsystem
  PRNDL_Flt : Lookup  InputValues=time  Table=PRNDL_Flt  LookUpMeth=Interpolation-Use End Values  OutDataTypeStr=int8
  Terminator : Terminator
  Terminator1 : Terminator
  tag scope: APP1_OOR_ON=global, APP2_OOR_ON=global, Brk_Flt=global, KeyPos_Flt_ON=global, Mismatch_APP_ON=global, PRNDL_Flt_ON=global
  wires:
  PRNDL_Flt/1 -> Override  PRNDL_Flt/1(In1)
  Override  KeyPos_Flt/1(Out1) -> [KeyPos_Flt_ON]
  BPP_Flt/1 -> Override  BPP_Flt/1(In1)
  APP1_OOR/1 -> Override  APP1_OOR/1(In1)
  Override  APP1_OOR/1(Out1) -> [APP1_OOR_ON]
  APP2_OOR/1 -> Override  APP2_OOR/1(In1)
  Override  APP2_OOR/1(Out1) -> [APP2_OOR_ON]
  Override  BPP_Flt/1(Out1) -> [Brk_Flt]
  Override  PRNDL_Flt/1(Out1) -> [PRNDL_Flt_ON]
  time/1 -> APP_Mismatch/1, APP2_OOR/1, PRNDL_Flt/1, KeyPos_Flt/1, BPP_Flt/1, APP1_OOR/1
  KeyPos_Flt/1 -> Override  KeyPos_Flt/1(In1)
  Override  APP_Mismatch/1(Out1) -> [Mismatch_APP_ON]  "APP_Mismatch"
  APP_Mismatch/1 -> Override  APP_Mismatch/1(In1)
  [APP1_OOR_ON] -> Terminator/1
  [PRNDL_Flt_ON] -> Terminator1/1

== system Clutchless_P2_Parallel_ETE/Sensors/Analog ==
  In1 : Inport
  Bus Creator : BusCreator  Inputs=4
  Bus Selector : BusSelector  OutputSignals=Driver_Signals.drv_APP1,Driver_Signals.drv_APP2,DC_mode,Driver_Signals.Sport_Mode_SW
  Data Type Conversion : DataTypeConversion
  Data Type Conversion1 : DataTypeConversion
  Data Type Conversion2 : DataTypeConversion
  Out1 : Outport
  wires:
  Data Type Conversion/1 -> Bus Creator/3  "DC_mode"
  Data Type Conversion1/1 -> Bus Creator/2  "Driver_APP2"
  Data Type Conversion2/1 -> Bus Creator/1  "Driver_APP1"
  In1/1 -> Bus Selector/1
  Bus Creator/1 -> Out1/1
  Bus Selector/3 -> Data Type Conversion/1  "<DC_mode>"
  Bus Selector/2 -> Data Type Conversion1/1  "<drv_APP2>"
  Bus Selector/1 -> Data Type Conversion2/1  "<drv_APP1>"
  Bus Selector/4 -> Bus Creator/4  "<Sport_Mode_SW>"

== system Clutchless_P2_Parallel_ETE/Sensors/CAN ==
  In1 : Inport
  Bus Creator : BusCreator  Inputs=3
  EBCAN : Subsystem
  HV_CAN : Subsystem
  VEH_CAN : Subsystem
  Out1 : Outport
  wires:
  In1/1 -> VEH_CAN/1(In1), EBCAN/1(In1), HV_CAN/1(In1)
  HV_CAN/1(Out1) -> Bus Creator/3  "fromHV_CAN"
  EBCAN/1(Out1) -> Bus Creator/2  "fromEBCAN"
  Bus Creator/1 -> Out1/1  "from_CAN"
  VEH_CAN/1(Out1) -> Bus Creator/1  "fromVEH_CAN"

== system Clutchless_P2_Parallel_ETE/Sensors/Digital ==
  In1 : Inport
  Bus Creator : BusCreator  Inputs=3
  Bus Selector : BusSelector  OutputSignals=Driver_Signals.SW_Regen_Disable,Driver_Signals.SW_Engine_ON,Driver_Signals.SW_CS_ON
  Data Type Conversion : DataTypeConversion
  Data Type Conversion1 : DataTypeConversion
  Data Type Conversion2 : DataTypeConversion
  Out1 : Outport
  wires:
  In1/1 -> Bus Selector/1
  Bus Selector/1 -> Data Type Conversion1/1  "<SW_Regen_Disable>"
  Bus Selector/2 -> Data Type Conversion/1  "<SW_Engine_ON>"
  Bus Selector/3 -> Data Type Conversion2/1  "<SW_CS_ON>"
  Data Type Conversion/1 -> Bus Creator/2  "SW_Engine_ON"
  Data Type Conversion2/1 -> Bus Creator/3  "SW_CS_ON"
  Data Type Conversion1/1 -> Bus Creator/1  "SW_Regen_Disable"
  Bus Creator/1 -> Out1/1  "Digital"

== system Clutchless_P2_Parallel_ETE/Actuators/CAN/EBCAN ==
  note: BMS_Antrieb
  note: ECM
  In1 : Inport
  Bus Creator : BusCreator  Inputs=7
  Bus Selector : BusSelector  OutputSignals=Controls.EngAppReq,Controls.EngOnReq,Controls.EngTrqCmd,Controls.ShftLvrPos,Controls.SysPwrMd
  Bus Selector1 : BusSelector  OutputSignals=BMS_CAN.ISO_Funktionaler_Req_All,BMS_CAN.ISO_Hybrid_01_Req
  ISO_Hybrid_01_Req : Subsystem
  PPEI_Platform_General_Status : Subsystem
  PPEI_Trans_General_Status_2 : Subsystem
  Out1 : Outport
  wires:
  Bus Creator/1 -> Out1/1
  PPEI_Platform_General_Status/1(Out1) -> Bus Creator/5
  Bus Selector/4 -> PPEI_Trans_General_Status_2/1(In1)  "<ShftLvrPos>"
  Bus Selector/5 -> PPEI_Platform_General_Status/1(In1)  "<SysPwrMd>"
  PPEI_Trans_General_Status_2/1(Out1) -> Bus Creator/4
  Bus Selector/3 -> Bus Creator/3  "<EngTrqCmd>"
  Bus Selector/2 -> Bus Creator/2  "<EngOnReq>"
  Bus Selector/1 -> Bus Creator/1  "<EngAppReq>"
  Bus Selector1/1 -> Bus Creator/6  "<ISO_Funktionaler_Req_All>"
  ISO_Hybrid_01_Req/1(Out1) -> Bus Creator/7
  Bus Selector1/2 -> ISO_Hybrid_01_Req/1(In1)  "<ISO_Hybrid_01_Req>"
  In1/1 -> Bus Selector/1, Bus Selector1/1

== system Clutchless_P2_Parallel_ETE/Actuators/CAN/HV_CAN ==
  In1 : Inport
  Bus Creator : BusCreator  Inputs=4
  Bus Creator1 : BusCreator  Inputs=1
  Bus Creator2 : BusCreator  Inputs=2
  Bus Creator3 : BusCreator  Inputs=5
  Bus Creator5 : BusCreator  Inputs=1
  Bus Selector : BusSelector  OutputSignals=BMS_CAN.MSG_HYB_01.MO_BMS_Sollmodus,Controls.Torque_Command,MCU_CAN.MCU_CAN.VCU_RequestedStateINV,OBC_CAN.NLG5_OC_COM,OBC_CAN.NLG5_OV_COM,OBC_CAN.NLG5_MC_MAX,OBC_CAN.NLG5_C_C_EL,OBC_CAN.NLG5_C_C_EN,MCU_CAN.DCDC_Out.DC_mode
  Data Type Conversion{,1..7} (8 alike) : DataTypeConversion
  Out1 : Outport
  wires:
  Bus Creator/1 -> Out1/1
  In1/1 -> Bus Selector/1
  Bus Selector/1 -> Data Type Conversion/1  "<MO_BMS_Sollmodus>"
  Data Type Conversion/1 -> Bus Creator1/1  "MO_BMS_Sollmodus"
  Bus Creator1/1 -> Bus Creator/1  "MSG_HYB_01"
  Bus Selector/2 -> Data Type Conversion1/1  "<Torque_Command>"
  Bus Selector/3 -> Data Type Conversion2/1  "<VCU_RequestedStateINV>"
  Bus Creator2/1 -> Bus Creator/2  "M192_Command_Message"
  Bus Selector/4 -> Data Type Conversion3/1  "<NLG5_OC_COM>"
  Bus Selector/5 -> Data Type Conversion4/1  "<NLG5_OV_COM>"
  Bus Selector/6 -> Data Type Conversion5/1  "<NLG5_MC_MAX>"
  Bus Selector/7 -> Data Type Conversion6/1  "<NLG5_C_C_EL>"
  Bus Selector/8 -> Data Type Conversion7/1  "<NLG5_C_C_EN>"
  Data Type Conversion1/1 -> Bus Creator2/1  "Torque_Command"
  Data Type Conversion2/1 -> Bus Creator2/2  "Inverter_Enable"
  Bus Creator3/1 -> Bus Creator/3  "NLG5_CTL"
  Data Type Conversion3/1 -> Bus Creator3/1  "NLG5_OC_COM"
  Data Type Conversion4/1 -> Bus Creator3/2  "NLG5_OV_COM"
  Data Type Conversion5/1 -> Bus Creator3/3  "NLG5_MC_MAX"
  Data Type Conversion6/1 -> Bus Creator3/4  "NLG5_C_C_EL"
  Data Type Conversion7/1 -> Bus Creator3/5  "NLG5_C_C_EN"
  Bus Selector/9 -> Bus Creator5/1  "<DC_mode>"
  Bus Creator5/1 -> Bus Creator/4  "DCDC"

== system Clutchless_P2_Parallel_ETE/Actuators/CAN/VEH_CAN ==
  note: TCM
  note: //*Divide the signals out of the Input by component before sending them in the TCM, EBCM etc blocks*//
  In1 : Inport
  BCM : Subsystem  Commented=on
  Bus Creator : BusCreator  Inputs=3
  Bus Creator1 : BusCreator  Inputs=1
  Bus Creator2 : BusCreator  Inputs=1
  Bus Creator3 : BusCreator  Inputs=1
  Bus Selector : BusSelector  OutputSignals=Controls.VehSpdAvgDrvn_kph,Controls.AccPos_Perc
  Data Type Conversion : DataTypeConversion
  Data Type Conversion1 : DataTypeConversion
  Data Type Conversion2 : DataTypeConversion
  EBCM : Subsystem  Commented=on
  Ground1 : Ground  Commented=on
  Ground2 : Ground  Commented=on
  Ground3 : Ground
  Ground4 : Ground  Commented=on
  ICCM : Subsystem  Commented=on
  Terminator : Terminator  Commented=on
  Terminator1 : Terminator  Commented=on
  Terminator2 : Terminator  Commented=on
  Out1 : Outport
  wires:
  ICCM/1(Out1) -> Terminator2/1  "HAct_to_ICCM"
  BCM/1(Out1) -> Terminator/1  "HAct_to_BCM"
  EBCM/1(Out1) -> Terminator1/1  "HAct_to_EBCM"
  Data Type Conversion/1 -> Bus Creator1/1  "VehSpdAvgDrvn"
  Bus Creator/1 -> Out1/1
  Ground1/1 -> EBCM/1(In1)
  Ground2/1 -> ICCM/1(In1)
  Bus Selector/2 -> Data Type Conversion1/1  "<AccPos_Perc>"
  Bus Selector/1 -> Data Type Conversion/1  "<VehSpdAvgDrvn_kph>"
  In1/1 -> Bus Selector/1
  Bus Creator1/1 -> Bus Creator/1  "PPEI_Vehicle_Speed_and_Distance"
  Data Type Conversion1/1 -> Bus Creator2/1  "AccActPos"
  Bus Creator2/1 -> Bus Creator/2  "PPEI_Engine_General_Status_1"
  Bus Creator3/1 -> Bus Creator/3  "ETEI_Engine_General_Status"
  Data Type Conversion2/1 -> Bus Creator3/1  "AccPdlPosPcntFullRng"
  Ground3/1 -> Data Type Conversion2/1
  Ground4/1 -> BCM/1(In1)

== system Clutchless_P2_Parallel_ETE/Camaro Plant Model/E-Machine/Clutch Temporary 1 ==
  In1 : Inport
  Constant : Constant  Value=0
  Memory : Memory
  Saturation : Saturate  UpperLimit=inf  LowerLimit=0
  Switch : Switch  Criteria=u2 > Threshold
  Out1 : Outport
  wires:
  Switch/1 -> Out1/1
  [cltch] -> Switch/2
  In1/1 -> Saturation/1
  Constant/1 -> Switch/3
  Memory/1 -> Switch/1
  Saturation/1 -> Memory/1

== system Clutchless_P2_Parallel_ETE/Camaro Plant Model/E-Machine/IMG Plant ==
  "In1 " : Inport
  voltage : Inport  Port=2
  MotShaftIn : Inport  Port=3
  SpdOut : Inport  Port=4
  " Actuators" : Subsystem
  Electric Machine : Subsystem
      mask Display:
      | image('Images\Motor.png')
      | color('red');
      | port_label('Input',1,'MotTrqCmd');
      | port_label('Input',2,'Volt');
      | port_label('Input',3,'ShaftIn');
      | port_label('Input',4,'SpdOut');
      | port_label('Output',1,'Crr')
      | port_label('Output',2,'SpdIn')
  Rate Transition7 : RateTransition  OutPortSampleTime=1
  Sensors : Subsystem
  To Workspace1 : ToWorkspace  VariableName=INV_ElectricMachineTemperature  SampleTime=-1
  Out1 : Outport
  current : Outport  Port=2
  MotShaftOut : Outport  Port=3
  SpdIn : Outport  Port=4
  tag scope: DirectionCommand=global, InverterEnabled=global, MotTrqCmd=global
  wires:
  voltage/1 -> Electric Machine/2(voltage2)
  ? -> [LockupCmd]
  [MotTrqCmd] -> Electric Machine/1(MotTrqCmd)
  Electric Machine/1(current) -> current/1
  Electric Machine/2(MotSpdIn1) -> SpdIn/1
  Electric Machine/3(mot_trq_out mot_inertia_out2) -> MotShaftOut/1
  [mot_trq_out] -> Sensors/2(In3)
  Sensors/1(Out1) -> Out1/1
  " Actuators"/1(MotTrqCmd) -> [MotTrqCmd]
  [mot_volt_in] -> Sensors/4(In5)
  "In1 "/1 -> " Actuators"/1(In1)
  [mot_crr_out] -> Sensors/3(In4)
  [mot_temp] -> Rate Transition7/1, Sensors/5(In6)
  " Actuators"/2(DirectionCommand) -> [DirectionCommand]
  " Actuators"/3(InverterEnabled) -> [InverterEnabled]
  [mcu_temp] -> Sensors/6(In1)
  SpdOut/1 -> Electric Machine/4(MotSpdOut)
  MotShaftIn/1 -> Electric Machine/3(mot_trq_in mot_inertia_in)
  [clt_plant_spd_in] -> Sensors/7(In7)
  [mot_spd_out] -> Sensors/1(In2)
  Rate Transition7/1 -> To Workspace1/1

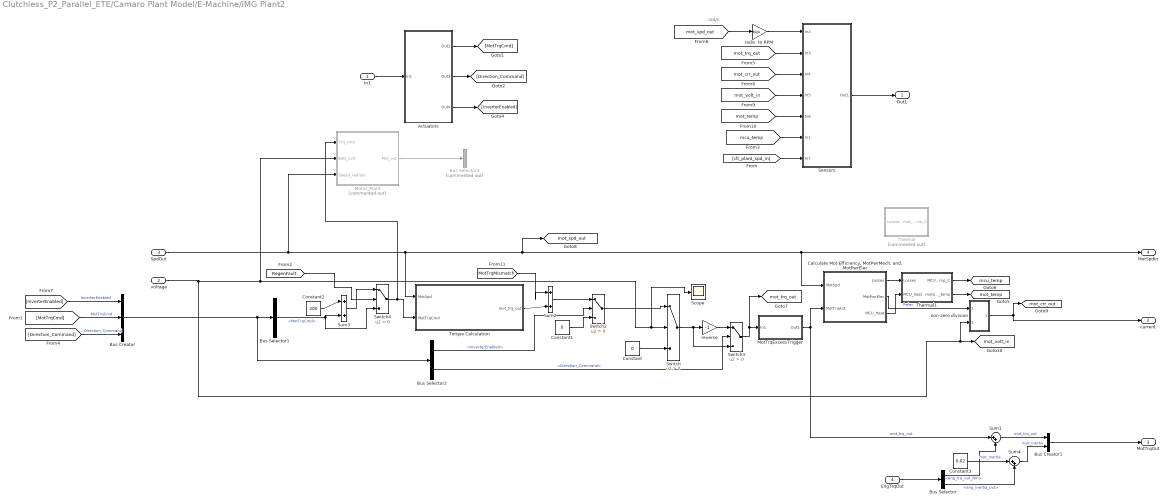
== system Clutchless_P2_Parallel_ETE/Camaro Plant Model/E-Machine/IMG Plant2 ==
  note: rad/s
  "In1 " : Inport
  voltage : Inport  Port=2
  SpdOut : Inport  Port=3
  EngTrqOut : Inport  Port=4
  " Actuators" : Subsystem
  Bus Creator : BusCreator  Inputs=3
  Bus Creator1 : BusCreator  Inputs=2
  Bus Selector : BusSelector  OutputSignals=eng_trq_out_Nm,eng_inertia_out
  Bus Selector1 : BusSelector  OutputSignals=MotTrqCmd
  Bus Selector2 : BusSelector  OutputSignals=InverterEnabled,Direction_Command
  Bus Selector3 : BusSelector  Commented=on  OutputSignals=Mot_current_A
  "Calculate Mot Efficiency, MotPwrMech, and, MotPwrElec" : Subsystem
  Constant : Constant  Value=0
  Constant1 : Constant  Value=0
  Constant2 : Constant  Value=200
  Constant3 : Constant  Value=0.02
  MotTrqExcessTrigger : Subsystem
  Motor_Plant : Subsystem  Commented=on
  Scope : Scope
  Sensors : Subsystem
  Sum{1..4} (4 alike) : Sum  Inputs=|++
  Switch{,2..4} (4 alike) : Switch  Criteria=u2 > Threshold
  Thermal : Subsystem  Commented=on
  Thermal1 : Subsystem
  Torque Calculation : Subsystem
  non-zero division : Subsystem
      mask Display: disp('divider \n I1/I2')
  rad/s  to RPM : Gain  Gain=30/pi
  reverse : Gain  Gain=-1
  Out1 : Outport
  current : Outport  Port=2
  MotTrqOut : Outport  Port=3
  MotSpdIn : Outport  Port=4
  tag scope: mcu_temp=global, mot_crr_out=global, mot_spd_out=global, mot_temp=global, mot_trq_out=global, mot_volt_in=global
  wires:
  Motor_Plant/1(Mot_out) -> Bus Selector3/1
  Bus Selector/1 -> Sum1/2  "<eng_trq_out_Nm>"
  Constant3/1 -> Sum4/1  "mot_inertia"
  Bus Selector/2 -> Sum4/2  "<eng_inertia_out>"
  Sum1/1 -> Bus Creator1/1  "mot_trq_out"
  EngTrqOut/1 -> Bus Selector/1
  Sum4/1 -> Bus Creator1/2  "mot_inertia"
  Bus Creator1/1 -> MotTrqOut/1
  voltage/1 -> Switch/2, Scope/1, Motor_Plant/2(Batt_volt), [mot_volt_in], non-zero division/2(In2)
  "Calculate Mot Efficiency, MotPwrMech, and, MotPwrElec"/2(MotPwrElec) -> non-zero division/1(In1)  "Pelec"
  MotTrqExcessTrigger/1(Out1) -> "Calculate Mot Efficiency, MotPwrMech, and, MotPwrElec"/2(MotTrqAct), Sum1/1  "mot_trq_out"
  "Calculate Mot Efficiency, MotPwrMech, and, MotPwrElec"/1(Losses) -> Thermal1/1(Losses)
  Constant/1 -> Switch/3
  "Calculate Mot Efficiency, MotPwrMech, and, MotPwrElec"/3(MCU_Heat) -> Thermal1/2(MCU_heat)
  Thermal1/2(motor_temp) -> [mot_temp]
  Switch/1 -> reverse/1, Switch3/3
  [MotTrqMismatch] -> Sum2/1
  Torque Calculation/1(mot_trq_out) -> Sum2/2
  Sum2/1 -> Switch2/1
  Bus Creator/1 -> Bus Selector1/1, Bus Selector2/1
  Bus Selector1/1 -> Sum3/2, Switch4/3  "<MotTrqCmd>"
  Bus Selector2/1 -> Switch2/2  "<InverterEnabled>"
  Constant1/1 -> Switch2/3
  Switch2/1 -> Switch/1
  Bus Selector2/2 -> Switch3/2  "<Direction_Command>"
  reverse/1 -> Switch3/1
  Switch3/1 -> MotTrqExcessTrigger/1(In1), [mot_trq_out]
  [RegenFault] -> Switch4/2
  Sum3/1 -> Switch4/1
  Switch4/1 -> Torque Calculation/2(MotTrqCmd), Motor_Plant/1(Trq_cmd)
  Constant2/1 -> Sum3/1
  Thermal1/1(MCU_temp_C) -> [mcu_temp]
  rad/s  to RPM/1 -> Sensors/1(In2)
  [mot_spd_out] -> rad/s  to RPM/1
  [MotTrqCmd] -> Bus Creator/2  "MotTrqCmd"
  [InverterEnabled] -> Bus Creator/1  "InverterEnabled"
  [Direction_Command] -> Bus Creator/3  "Direction_Command"
  " Actuators"/3(Out4) -> [InverterEnabled]
  " Actuators"/2(Out3) -> [Direction_Command]
  [clt_plant_spd_in] -> Sensors/7(In7)
  [mcu_temp] -> Sensors/6(In1)
  non-zero division/1(Out1) -> [mot_crr_out], current/1
  SpdOut/1 -> "Calculate Mot Efficiency, MotPwrMech, and, MotPwrElec"/1(MotSpd), MotSpdIn/1, [mot_spd_out], Torque Calculation/1(MotSpd), Motor_Plant/3(Speed_rad/sec)
  [mot_trq_out] -> Sensors/2(In3)
  Sensors/1(Out1) -> Out1/1
  " Actuators"/1(Out2) -> [MotTrqCmd]
  [mot_volt_in] -> Sensors/4(In5)
  "In1 "/1 -> " Actuators"/1(In1)
  [mot_crr_out] -> Sensors/3(In4)
  [mot_temp] -> Sensors/5(In6)
